simulink model "Ass2_extraB_LQR"  (R2024b)
settings: Solver=FixedStepAuto  StartTime=0.0  StopTime=inf  FixedStep=1/f_sim  RelTol=1e-3
values from neighbouring files (symbols this model uses):
  f_cmd = 100    [Main_ass2_extraB_LQR.m]
  f_odom = 100    [Main_ass2_extraB_LQR.m]
  N_way = length(x_way)    [Main_Optimisation.m]    (also in Main_ass2_extraB_LQR.m; optimal_data.mat = 11)
  toll_dist = 0.6    [Main_ass2_extraB_LQR.m]
  v_max = 0.5    [Main_Optimisation.m]    (also in Main_ass2_extraB_LQR.m = 0.6; optimise.m = param.v_max)
  v_min = 0    [Main_Optimisation.m]    (also in Main_ass2_extraB_LQR.m; optimise.m = param.v_min)
  w_max = 1    [Main_Optimisation.m]    (also in Main_ass2_extraB_LQR.m; optimise.m = param.w_max)
  w_min = -1    [Main_Optimisation.m]    (also in Main_ass2_extraB_LQR.m; optimise.m = param.w_min)
  waypoints = [x_way' y_way' orient_way']    [Main_Optimisation.m]    (also in Main_ass2_extraB_LQR.m; optimal_data.mat = [0 5 5 -5 -5 0 3 -3 0 3 0 0 ... (33 elements, 11x3)])
undefined symbols (not defined in the file or in its folder): Angular, Linear
libraries: robotlib x3, simulink x3, hdlsllib x1
settings Model: Creator=vise  LastModifiedBy=vise
settings OptimizationCC: DefaultParameterBehavior=Inlined  EnhancedBackFolding=on  PassReuseOutputArgsAs=Individual arguments  ZeroExternalMemoryAtStartup=off  ZeroInternalMemoryAtStartup=off  MaxStackSize=64  OptimizeBlockOrder=speed  DifferentSizesBufferReuse=on  OptimizationCustomize=off  EfficientTunableParamExpr=on
settings DebuggingCC: ParameterTunabilityLossMsg=error
settings HardwareCC: ProdBitPerPointer=32  ProdBitPerSizeT=32  ProdBitPerPtrDiffT=32  ProdLargestAtomicFloat=None  ProdIntDivRoundTo=Undefined  ProdEndianess=Unspecified  ProdWordSize=32  ProdHWDeviceType=Generic->Unspecified (assume 32-bit Generic)  UseEmbeddedCoderFeatures=off
settings SFSimCC: MATLABDynamicMemAlloc=off
settings RTWCC: Description=Embedded Coder  SystemTargetFile=ert.tlc  HardwareBoard=Robot Operating System (ROS)  TLCOptions="-aInlineSetEventsForThisBaseRateFcn=TLC_FALSE -aSuppressMultiTaskScheduler=TLC_FALSE  -aRateBasedStepFcn=0"  TemplateMakefile=ert_default_tmf  Toolchain=Catkin  TargetLang=C++
settings CodeAppCC: ForceParamTrailComments=on  IgnoreCustomStorageClasses=off  OperatorAnnotations=on  SimulinkDataObjDesc=on  SFDataObjDesc=on  InsertBlockDesc=on
settings ERTTargetCC: SupportNonInlinedSFcns=on

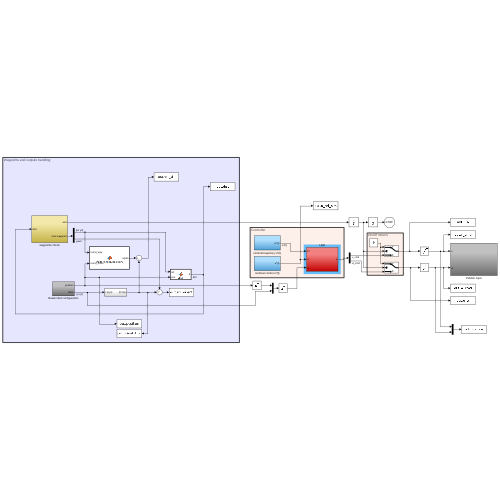
[thumbnail: Simulink's stored preview of the top-level diagram]
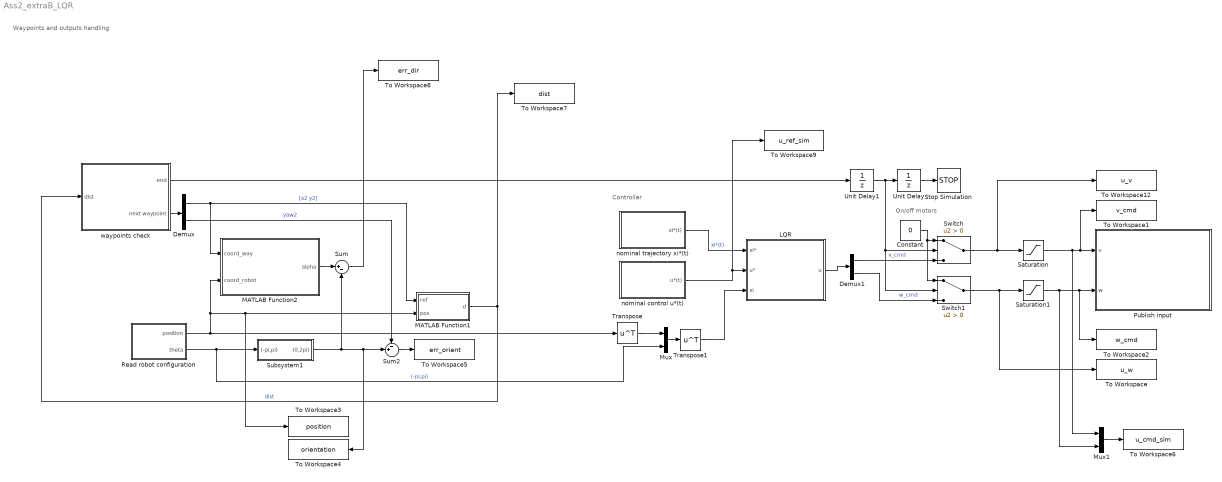
== system Ass2_extraB_LQR ==
  note: Controller
  note: Waypoints and outputs handling
  note: On/off motors
  Constant : Constant  Value=0
  Demux : Demux  Outputs=2
  Demux1 : Demux  Outputs=2
  LQR : Subsystem
  MATLAB Function1 : MATLAB Function  TreatAsAtomicUnit=on
  MATLAB Function2 : MATLAB Function  TreatAsAtomicUnit=on
  Mux : Mux  Inputs=2
  Mux1 : Mux  Inputs=2
  Publish input : Subsystem
  Read robot configuration : Subsystem
  Saturation : Saturate  UpperLimit=v_max  LowerLimit=v_min
  Saturation1 : Saturate  UpperLimit=w_max  LowerLimit=w_min
  Stop Simulation : Stop
  Subsystem1 : Subsystem
  Sum : Sum  Inputs=|+-
  Sum2 : Sum  Inputs=-+|
  Switch : Switch  Criteria=u2 > Threshold  SaturateOnIntegerOverflow=off  InputSameDT=off
  Switch1 : Switch  Criteria=u2 > Threshold  SaturateOnIntegerOverflow=off  InputSameDT=off
  To Workspace : ToWorkspace  VariableName=u_w  SampleTime=-1
      settings: Save2DSignal=2-D array (concatenate along first dimension)
  To Workspace1 : ToWorkspace  VariableName=v_cmd  SampleTime=-1
      settings: Save2DSignal=2-D array (concatenate along first dimension)
  To Workspace12 : ToWorkspace  VariableName=u_v  SampleTime=-1
      settings: Save2DSignal=2-D array (concatenate along first dimension)
  To Workspace2 : ToWorkspace  VariableName=w_cmd  SampleTime=-1
      settings: Save2DSignal=2-D array (concatenate along first dimension)
  To Workspace3 : ToWorkspace  VariableName=position  SampleTime=-1
      settings: Save2DSignal=2-D array (concatenate along first dimension)
  To Workspace4 : ToWorkspace  VariableName=orientation  SampleTime=-1
      settings: Save2DSignal=2-D array (concatenate along first dimension)
  To Workspace5 : ToWorkspace  VariableName=err_orient  SampleTime=-1
      settings: Save2DSignal=2-D array (concatenate along first dimension)
  To Workspace6 : ToWorkspace  VariableName=u_cmd_sim  SampleTime=-1
      settings: Save2DSignal=2-D array (concatenate along first dimension)
  To Workspace7 : ToWorkspace  VariableName=dist  SampleTime=-1
      settings: Save2DSignal=2-D array (concatenate along first dimension)
  To Workspace8 : ToWorkspace  VariableName=err_dir  SampleTime=-1
      settings: Save2DSignal=2-D array (concatenate along first dimension)
  To Workspace9 : ToWorkspace  VariableName=u_ref_sim  SampleTime=-1
      settings: Save2DSignal=2-D array (concatenate along first dimension)
  Transpose : Math  Operator=transpose
  Transpose1 : Math  Operator=transpose
  Unit Delay : UnitDelay  SampleTime=3  HasFrameUpgradeWarning=on
  Unit Delay1 : UnitDelay  SampleTime=0.5  HasFrameUpgradeWarning=on
  nominal control u*(t) : Subsystem
  nominal trajectory xi*(t) : Subsystem
  waypoints check : Subsystem
  wires:
  Demux/1 -> MATLAB Function2/1(coord_way), MATLAB Function1/1(ref)  "[x2 y2]"
  MATLAB Function1/1(d) -> waypoints check/1(dist), To Workspace7/1  "dist"
  MATLAB Function2/1(alpha) -> Sum/1
  Demux/2 -> Sum2/1  "yaw2"
  Read robot configuration/2(theta) -> Mux/2, Subsystem1/1((-pi,pi))  "(-pi,pi)"
  waypoints check/2(next waypoint) -> Demux/1
  waypoints check/1(end) -> Unit Delay1/1
  Switch/1 -> Saturation/1, To Workspace12/1
  Constant/1 -> Switch1/1, Switch/1
  Sum2/1 -> To Workspace5/1
  Sum/1 -> To Workspace8/1
  Switch1/1 -> Saturation1/1, To Workspace/1
  LQR/1(u) -> Demux1/1
  nominal control u*(t)/1(u*(t)) -> To Workspace9/1, LQR/2(u*)
  Read robot configuration/1(position) -> Transpose/1, MATLAB Function2/2(coord_robot), To Workspace3/1, MATLAB Function1/2(pos)
  Transpose/1 -> Mux/1
  Mux/1 -> Transpose1/1
  Subsystem1/1((0,2pi)) -> To Workspace4/1, Sum2/2, Sum/2
  Saturation/1 -> Mux1/1, To Workspace1/1, Publish input/1(v)
  Saturation1/1 -> Mux1/2, To Workspace2/1, Publish input/2(w)
  Demux1/2 -> Switch1/3  "w_cmd"
  Unit Delay/1 -> Stop Simulation/1
  Demux1/1 -> Switch/3  "v_cmd"
  Mux1/1 -> To Workspace6/1
  Unit Delay1/1 -> Switch1/2, Switch/2, Unit Delay/1
  Transpose1/1 -> LQR/3(xi)
  nominal trajectory xi*(t)/1(xi*(t)) -> LQR/1(xi*)  "xi*(t)"

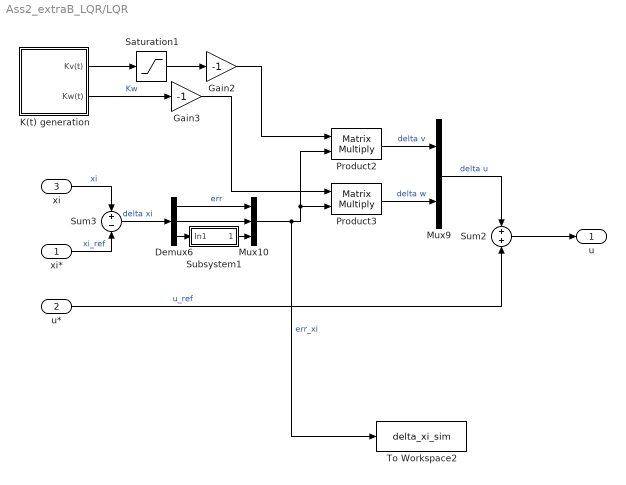
== system Ass2_extraB_LQR/LQR ==
  xi* : Inport
  u* : Inport  Port=2
  xi : Inport  Port=3
  Demux6 : Demux  Outputs=3
  Gain2 : Gain  Gain=-1
  Gain3 : Gain  Gain=-1
  K(t) generation : Subsystem
  Mux10 : Mux  Inputs=3
  Mux9 : Mux  Inputs=2
  Product2 : Product  Multiplication=Matrix(*)
  Product3 : Product  Multiplication=Matrix(*)
  Saturation1 : Saturate  UpperLimit=0  LowerLimit=-inf
  Subsystem1 : Subsystem
  Sum2 : Sum  Inputs=+|+
  Sum3 : Sum  Inputs=+|-
  To Workspace2 : ToWorkspace  VariableName=delta_xi_sim  SampleTime=-1
  u : Outport
  wires:
  u*/1 -> Sum2/2  "u_ref"
  Subsystem1/1(Out1) -> Mux10/3
  Demux6/2 -> Mux10/2
  Product2/1 -> Mux9/1  "delta v"
  xi*/1 -> Sum3/2  "xi_ref"
  xi/1 -> Sum3/1  "xi"
  K(t) generation/1(Kv(t)) -> Saturation1/1
  Gain2/1 -> Product2/1
  Mux9/1 -> Sum2/1  "delta u"
  Mux10/1 -> To Workspace2/1, Product3/2, Product2/2  "err_xi"
  Demux6/1 -> Mux10/1  "err"
  Gain3/1 -> Product3/1
  Sum2/1 -> u/1
  Demux6/3 -> Subsystem1/1(In1)
  Product3/1 -> Mux9/2  "delta w"
  K(t) generation/2(Kw(t)) -> Gain3/1  "Kw"
  Sum3/1 -> Demux6/1  "delta xi"
  Saturation1/1 -> Gain2/1

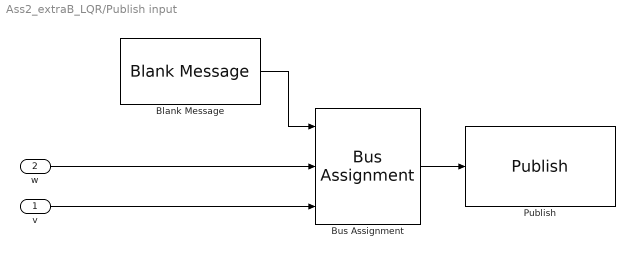
== system Ass2_extraB_LQR/Publish input ==
  v : Inport
  w : Inport  Port=2
  Blank Message : robotlib/Blank Message  messageClass=Message  entityType=geometry_msgs/Twist  messageType=geometry_msgs/Twist  SampleTime=1/f_cmd  legacyBusStruct=off
  Bus Assignment : BusAssignment  AssignedSignals=Angular.Z,Linear.X
  Publish : robotlib/Publish  topicSource=Select from ROS network  topic=/cmd_vel  messageType=geometry_msgs/Twist  legacyBusStruct=off  messageQueueLength=1
  wires:
  Bus Assignment/1 -> Publish/1
  Blank Message/1 -> Bus Assignment/1
  w/1 -> Bus Assignment/2
  v/1 -> Bus Assignment/3

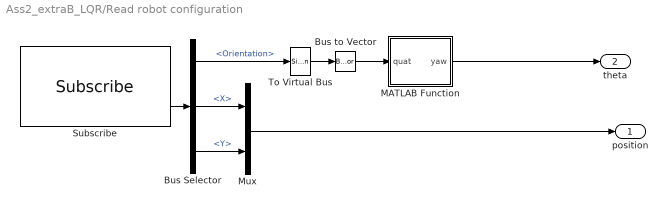
== system Ass2_extraB_LQR/Read robot configuration ==
  Bus Selector : BusSelector  OutputSignals=Pose.Pose.Orientation,Pose.Pose.Position.X,Pose.Pose.Position.Y
  Bus to Vector : BusToVector
  MATLAB Function : MATLAB Function  TreatAsAtomicUnit=on
  Mux : Mux  Inputs=2
  Subscribe : robotlib/Subscribe  topicSource=Select from ROS network  topic=/odom  messageType=nav_msgs/Odometry  SampleTime=1/f_odom  legacyBusStruct=off  messageQueueLength=1
  To Virtual Bus : SignalConversion  ConversionOutput=Virtual bus  OverrideOpt=off
  position : Outport
  theta : Outport  Port=2
  wires:
  Bus to Vector/1 -> MATLAB Function/1(quat)
  Mux/1 -> position/1
  Bus Selector/1 -> To Virtual Bus/1  "<Orientation>"
  Bus Selector/2 -> Mux/1  "<X>"
  To Virtual Bus/1 -> Bus to Vector/1
  Subscribe/2 -> Bus Selector/1
  Bus Selector/3 -> Mux/2  "<Y>"
  MATLAB Function/1(yaw) -> theta/1

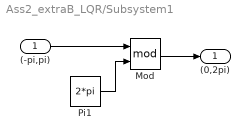
== system Ass2_extraB_LQR/Subsystem1 ==
  (-pi,pi) : Inport
  Mod : Math  Operator=mod
  Pi1 : Constant  Value=2*pi  OutDataTypeStr=Inherit: Inherit via back propagation
  (0,2pi) : Outport
  wires:
  (-pi,pi)/1 -> Mod/1
  Pi1/1 -> Mod/2
  Mod/1 -> (0,2pi)/1

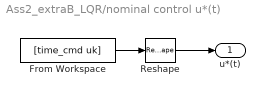
== system Ass2_extraB_LQR/nominal control u*(t) ==
  From Workspace : FromWorkspace  VariableName=[time_cmd uk]  OutputAfterFinalValue=Holding final value
  Reshape : Reshape  OutputDimensionality=Column vector (2-D)
  u*(t) : Outport
  wires:
  Reshape/1 -> u*(t)/1
  From Workspace/1 -> Reshape/1

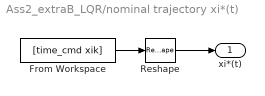
== system Ass2_extraB_LQR/nominal trajectory xi*(t) ==
  From Workspace : FromWorkspace  VariableName=[time_cmd xik]  OutputAfterFinalValue=Holding final value
  Reshape : Reshape  OutputDimensionality=Column vector (2-D)
  xi*(t) : Outport
  wires:
  From Workspace/1 -> Reshape/1
  Reshape/1 -> xi*(t)/1

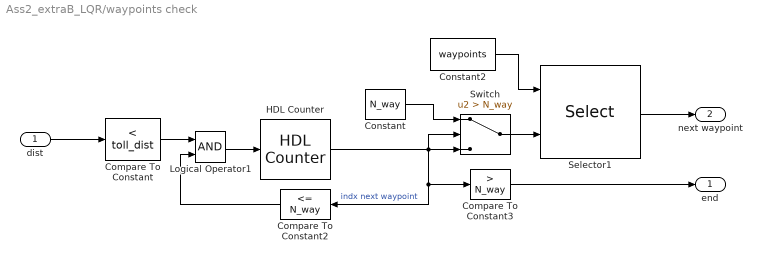
== system Ass2_extraB_LQR/waypoints check ==
  dist : Inport
  Compare To Constant : simulink/Logic and Bit Operations/Compare To Constant  relop=<  const=toll_dist  OutDataTypeStr=boolean
  Compare To Constant2 : simulink/Logic and Bit Operations/Compare To Constant  relop=<=  const=N_way  OutDataTypeStr=boolean
  Compare To Constant3 : simulink/Logic and Bit Operations/Compare To Constant  relop=>  const=N_way  OutDataTypeStr=boolean
  Constant : Constant  Value=N_way
  Constant2 : Constant  Value=waypoints
  HDL Counter : hdlsllib/Sources/HDL Counter  CountType=Count limited  CountInit=1  CountStep=1  CountMax=N_way+1  CountFromType=Initial value  CountFrom=1  CountResetPort=off  CountLoadPort=off  CountEnbPort=on  CountDirPort=off  CountHitOutputPort=off  CountDataType=Unsigned  CountWordLen=8  CountFracLen=0  CountSampTime=1
  Logical Operator1 : Logic  AllPortsSameDT=off  OutDataTypeStr=boolean
  Selector1 : Selector  NumberOfDimensions=2  InputPortWidth=3  IndexOptions=Index vector (port),Select all  Indices=[1 3],[1 2]  OutputSizes=1,1
  Switch : Switch  Criteria=u2 > Threshold  Threshold=N_way  SaturateOnIntegerOverflow=off  InputSameDT=off
  end : Outport
  next waypoint : Outport  Port=2
  wires:
  HDL Counter/1 -> Compare To Constant3/1, Compare To Constant2/1, Switch/3, Switch/2  "indx next waypoint"
  Compare To Constant/1 -> Logical Operator1/1
  dist/1 -> Compare To Constant/1
  Selector1/1 -> next waypoint/1
  Constant2/1 -> Selector1/1
  Logical Operator1/1 -> HDL Counter/1
  Compare To Constant2/1 -> Logical Operator1/2
  Switch/1 -> Selector1/2
  Constant/1 -> Switch/1
  Compare To Constant3/1 -> end/1

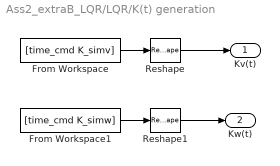
== system Ass2_extraB_LQR/LQR/K(t) generation ==
  From Workspace : FromWorkspace  VariableName=[time_cmd K_simv]  OutputAfterFinalValue=Holding final value
  From Workspace1 : FromWorkspace  VariableName=[time_cmd K_simw]  OutputAfterFinalValue=Holding final value
  Reshape : Reshape  OutputDimensionality=Row vector (2-D)
  Reshape1 : Reshape  OutputDimensionality=Row vector (2-D)
  Kv(t) : Outport
  Kw(t) : Outport  Port=2
  wires:
  From Workspace/1 -> Reshape/1
  Reshape/1 -> Kv(t)/1
  From Workspace1/1 -> Reshape1/1
  Reshape1/1 -> Kw(t)/1

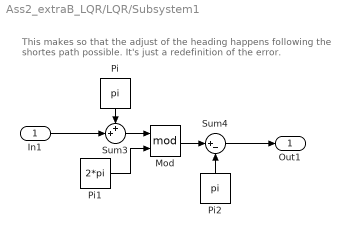
== system Ass2_extraB_LQR/LQR/Subsystem1 ==
  note: This makes so that the adjust of the heading happens following
      | the shortes path possible. It's just a redefinition of the error.
  In1 : Inport
  Mod : Math  Operator=mod
  Pi : Constant  Value=pi  OutDataTypeStr=Inherit: Inherit via back propagation
  Pi1 : Constant  Value=2*pi  OutDataTypeStr=Inherit: Inherit via back propagation
  Pi2 : Constant  Value=pi  OutDataTypeStr=Inherit: Inherit via back propagation
  Sum3 : Sum  Inputs=++|
  Sum4 : Sum  Inputs=|+-
  Out1 : Outport
  wires:
  Sum4/1 -> Out1/1
  In1/1 -> Sum3/2
  Pi2/1 -> Sum4/2
  Pi/1 -> Sum3/1
  Pi1/1 -> Mod/2
  Sum3/1 -> Mod/1
  Mod/1 -> Sum4/1

== matlab function Ass2_extraB_LQR/Read robot configuration/MATLAB Function ==
  data: quat input; yaw output
function yaw=quat2yaw(quat)

q=zeros(1,4);

q(1)=quat(1);
q(2)=quat(2);
q(3)=quat(3);
q(4)=quat(4);

eul=quat2eul(q);

yaw=eul(3);

end

== matlab function Ass2_extraB_LQR/MATLAB Function2 ==
  data: coord_way input; alpha output; coord_robot input
function alpha=ReferenceDirection(coord_way,coord_robot)

% computes the direction (angle wrt positive x axis,
% counterclockwise) between two inputed points [x1 y1 ; x2 y2] 

x1=coord_robot(1);
y1=coord_robot(2);
x2=coord_way(1);
y2=coord_way(2);

alpha=atan2((y2-y1),(x2-x1)); % (-pi,pi)

alpha=mod(alpha,2*pi); % (0,2pi)

end

== matlab function Ass2_extraB_LQR/MATLAB Function1 ==
  data: ref input; d output; pos input
function d=dist(ref,pos)

% computes the distance between two points (x1,y1) and (x2,y2)

x_ref=ref(1);
y_ref=ref(2);
x_pos=pos(1);
y_pos=pos(2);

d=sqrt((x_ref-x_pos)^2+(y_ref-y_pos)^2);

end
